simulink library "CTRL_TRGT_SADES"  (R2023b)
settings: Solver=VariableStepAuto  StartTime=0.0  StopTime=10.0  RelTol=1e-3
undefined symbols (not defined in the file): p_TirCorStiRe_Nprad
libraries: VUT_lib x1
settings Model: Creator=blatak  LastModifiedBy=blatak

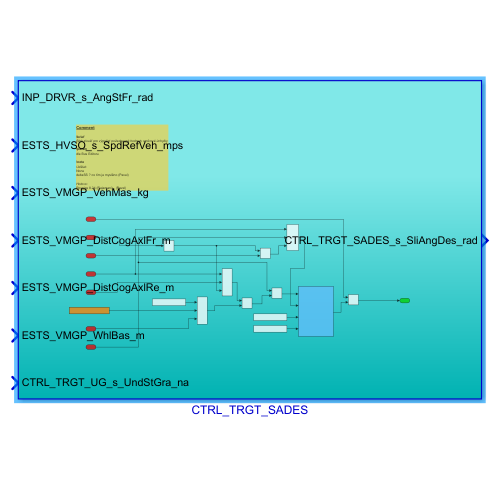
[thumbnail: Simulink's stored preview of the top-level diagram]
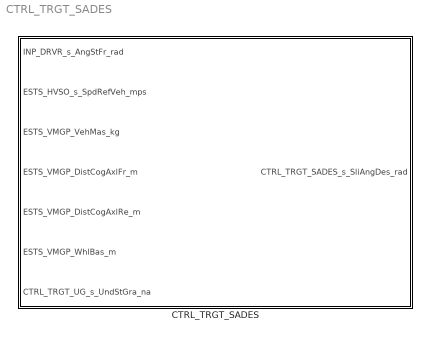
== system CTRL_TRGT_SADES ==
  CTRL_TRGT_SADES : Subsystem

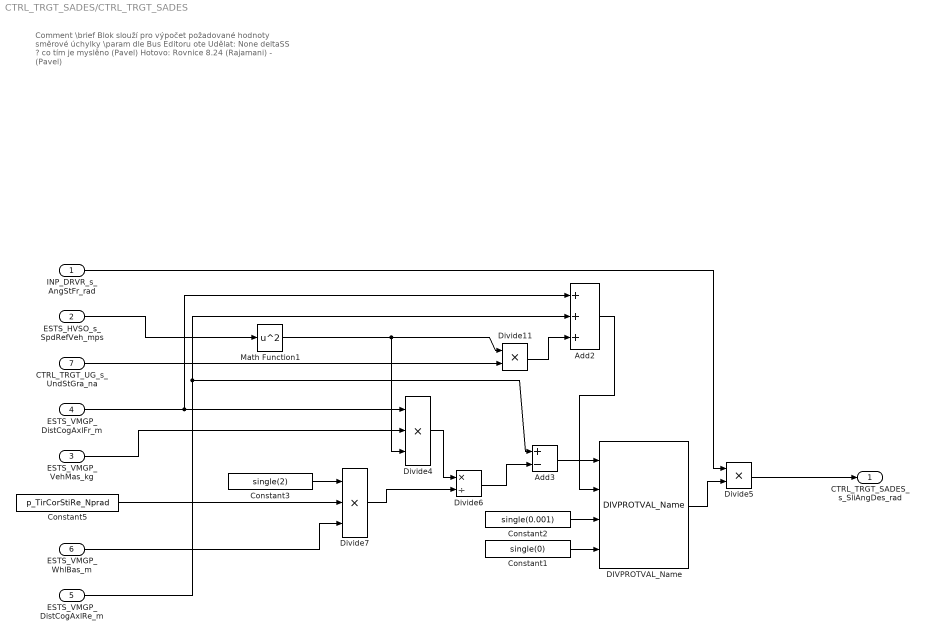
== system CTRL_TRGT_SADES/CTRL_TRGT_SADES ==
  note: Comment
      |
      | \brief
      | Blok slouží pro výpočet požadované hodnoty směrové úchylky
      |
      | \param
      | dle Bus Editoru
      |
      | \note
      | Udělat:
      | None
      | deltaSS ? co tím je myslěno (Pavel)
      |
      | Hotovo:
      | Rovnice 8.24 (Rajamani) - (Pavel)
  INP_DRVR_s_AngStFr_rad : Inport
  ESTS_HVSO_s_SpdRefVeh_mps : Inport  Port=2
  ESTS_VMGP_VehMas_kg : Inport  Port=3
  ESTS_VMGP_DistCogAxlFr_m : Inport  Port=4
  ESTS_VMGP_DistCogAxlRe_m : Inport  Port=5
  ESTS_VMGP_WhlBas_m : Inport  Port=6
  CTRL_TRGT_UG_s_UndStGra_na : Inport  Port=7
  Add2 : Sum  Inputs=+++
  Add3 : Sum  Inputs=+-
  Constant1 : Constant  Value=single(0)
  Constant2 : Constant  Value=single(0.001)
  Constant3 : Constant  Value=single(2)
  Constant5 : Constant  Value=p_TirCorStiRe_Nprad
  DIVPROTVAL_Name : VUT_lib/DIVPROTVAL_Name  SystemSampleTime=-1  VariantActivationTime=update diagram  AllowFlexibleInterface=on  Latency=0  AutoFrameSizeCalculation=off
  Divide11 : Product  Inputs=**
  Divide4 : Product  Inputs=***
  Divide5 : Product  Inputs=**
  Divide6 : Product  Inputs=*/
  Divide7 : Product  Inputs=***
  Math Function1 : Math  Operator=square
  CTRL_TRGT_SADES_s_SliAngDes_rad : Outport
  wires:
  Divide6/1 -> Add3/2
  INP_DRVR_s_AngStFr_rad/1 -> Divide5/1
  Add2/1 -> DIVPROTVAL_Name/2
  ESTS_VMGP_WhlBas_m/1 -> Divide7/3
  Divide5/1 -> CTRL_TRGT_SADES_s_SliAngDes_rad/1
  DIVPROTVAL_Name/1 -> Divide5/2
  Divide4/1 -> Divide6/1
  ESTS_VMGP_DistCogAxlFr_m/1 -> Add2/1, Divide4/1
  Divide11/1 -> Add2/3
  CTRL_TRGT_UG_s_UndStGra_na/1 -> Divide11/2
  ESTS_VMGP_DistCogAxlRe_m/1 -> Add2/2, Add3/1
  Math Function1/1 -> Divide4/3, Divide11/1
  Divide7/1 -> Divide6/2
  Add3/1 -> DIVPROTVAL_Name/1
  ESTS_HVSO_s_SpdRefVeh_mps/1 -> Math Function1/1
  ESTS_VMGP_VehMas_kg/1 -> Divide4/2
  Constant3/1 -> Divide7/1
  Constant5/1 -> Divide7/2
  Constant1/1 -> DIVPROTVAL_Name/4
  Constant2/1 -> DIVPROTVAL_Name/3
